simulink model "a6_1_solving_mathematical_equations"  (R2018a)
settings: Solver=VariableStepAuto  StartTime=0.0  StopTime=10.0  RelTol=1e-3
settings Model: Creator=r0x6f736f646f  LastModifiedBy=r0x6f736f646f

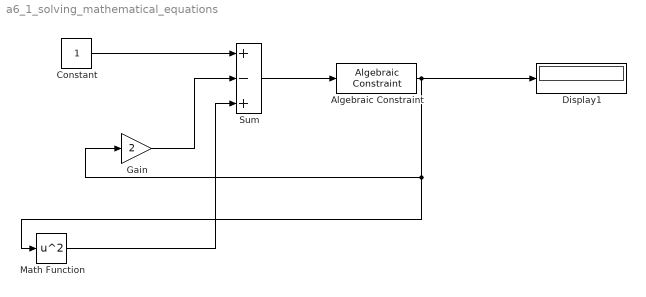
== system a6_1_solving_mathematical_equations ==
  Algebraic Constraint : AlgebraicConstraint
  Constant : Constant
  Display1 : Display
  Gain : Gain  Gain=2
  Math Function : Math  Operator=square  SaturateOnIntegerOverflow=on
  Sum : Sum  Inputs=+-+
  wires:
  Algebraic Constraint/1 -> Math Function/1, Gain/1, Display1/1
  Constant/1 -> Sum/1
  Sum/1 -> Algebraic Constraint/1
  Gain/1 -> Sum/2
  Math Function/1 -> Sum/3
